simulink model "Filter"  (R2020b)
settings: Solver=VariableStepAuto  StartTime=0.0  StopTime=10.0  RelTol=1e-3
settings Model: Creator=JAGRUTI SHINDE  LastModifiedBy=JAGRUTI SHINDE
settings DataIOCC: SaveOutput=off  SaveTime=off

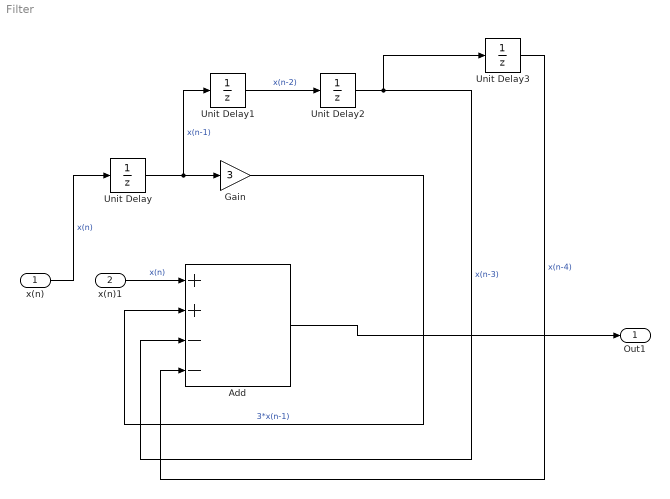
== system Filter ==
  x(n) : Inport  OutDataTypeStr=double  PortDimensions=1  SampleTime=0
  x(n)1 : Inport  Port=2  OutDataTypeStr=double  PortDimensions=1  SampleTime=0
  Add : Sum  Inputs=++--
  Gain : Gain  Gain=3
  Unit Delay{,1..3} (4 alike) : UnitDelay  SampleTime=-1  HasFrameUpgradeWarning=on
  Out1 : Outport  OutDataTypeStr=double  PortDimensions=1  SampleTime=0
  wires:
  x(n)1/1 -> Add/1  "x(n)"
  Unit Delay2/1 -> Add/3, Unit Delay3/1  "x(n-3)"
  Unit Delay3/1 -> Add/4  "x(n-4)"
  Unit Delay/1 -> Gain/1, Unit Delay1/1  "x(n-1)"
  Add/1 -> Out1/1
  Gain/1 -> Add/2  "3*x(n-1)"
  Unit Delay1/1 -> Unit Delay2/1  "x(n-2)"
  x(n)/1 -> Unit Delay/1  "x(n)"
